simulink model "Pitoni_02"  (R2022b)
settings: Solver=VariableStepAuto  StartTime=0.0  StopTime=10  RelTol=1e-3
settings Model: Creator=Stefano  LastModifiedBy=stefanopanzieri
settings SolverCC: AlgebraicLoopSolver=TrustRegion
settings OptimizationCC: ReuseModelBlockBuffer=on
settings DebuggingCC: UnconnectedInputMsg=warning  UnconnectedOutputMsg=warning  UnconnectedLineMsg=warning
settings ModelReferenceCC: EnableRefExpFcnMdlSchedulingChecks=on
settings SFSimCC: CustomCodeUndefinedFunction=UseInterfaceOnly
settings RTWCC: DLArmComputeVersion=19.05

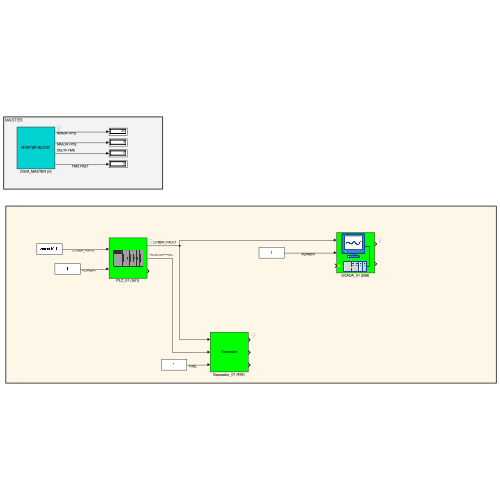
[thumbnail: Simulink's stored preview of the top-level diagram]
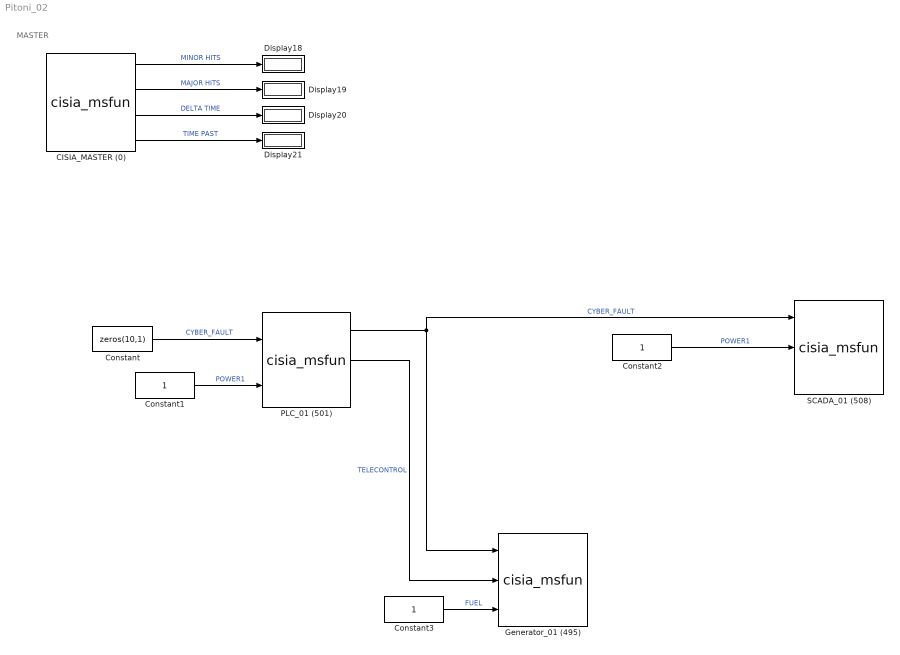
== system Pitoni_02 ==
  note: MASTER
  CISIA_MASTER (0) : M-S-Function  FunctionName=cisia_msfun  Parameters=Parameter1, Parameter2, Parameter3, resources, Parameter4, Parameter5, Parameter6, Parameter7, Parameter8, Parameter9,Parameter11  mask(S-function:msfcn_unit_delay){Parameter1='CISIA_MASTER', Parameter2=1, Parameter3='Pitoni', resources=off, Parameter4=on, Parameter5=off, Parameter6=off, Parameter7=off, Parameter8=0.001, Parameter9=off, Parameter11=on}
      mask prompts: Parameter1 "entity name"; Parameter2 "sampling time"; Parameter3 "project"; resources "Save status at each major hit"; Parameter4 "Show Operative Levels with colors"; Parameter5 "Load Entities from file"; Parameter6 "Load Start from Mask"; Parameter7 "Real Time"; Parameter8 "Real Time Hit (sec)"; Parameter9 "Skip saving"; Parameter11 "Show unconnected"
      mask help: This is a level-2 MATLAB file S-function which demonstrates CISIA entity
      mask Display: disp('MASTER BLOCK')
  Constant : Constant  Value=zeros(10,1)
  Constant1 : Constant
  Constant2 : Constant
  Constant3 : Constant
  Display{18..21} (4 alike) : Display
  Generator_01 (495) : M-S-Function  FunctionName=cisia_msfun  Parameters=Parameter1, Parameter2, Parameter3, resources, Parameter10, codeupdate, step_received, step_computed, dynamic_computed, step_sended, id_entity, id_project, id_type, name_type, color  mask(S-function:msfcn_unit_delay){Parameter1='Generator_01', Parameter2=1, Parameter3='', resources=|, Parameter10=off, codeupdate=off, step_received=|, step_computed=, dynamic_computed=, step_sended=|, id_entity=495, id_project=44, id_type=117, name_type=Generator, color=#FFFFFF}
      mask resources=|
      | *** INPUT RESOURCES ***
      | NUM_INPUTS 3
      | CYBER_FAULT (10)
      | TELECONTROL (1)
      | FUEL (1)
      |
      | *** STATE VARIABLES ***
      | NUM_VARIABLES 14
      | Operative_Level(NUMERIC)(1)(1)
      | Dos_attack(NUMERIC)(1)(0)
      | MITM_attack(NUMERIC)(1)(0)
      | Virus_Attack(NUMERIC)(1)(0)
      | Port_Scan_Attack(NUMERIC)(1)(0)
      | Cyber_Fault(NUMERIC_ARRAY)(10)(0  0  0  0  0  0  0  0  0  0)
      | BGP_hijacking(NUMERIC)(1)(0)
      | Mechanical_Fault(NUMERIC)(1)(0)
      | BotNet_Attack(NUMERIC)(1)(0)
      | Data_Corruption(NUMERIC)(1)(0)
      | SW_Change(NUMERIC)(1)(0)
      | Config_Change(NUMERIC)(1)(0)
      | Port_Saturation(NUMERIC)(1)(0)
      | Control_Fault(NUMERIC)(1)(0)
      |
      | *** OUTPUT RESOURCES ***
      | NUM_OUTPUTS 3
      | CYBER_FAULT (10)
      | POWER1 (1)
      | GENERATOR_QoS (1)
      mask step_received=|
      | Cyber_Fault=max(CYBER_FAULT, transpose([Dos_attack MITM_attack Virus_Attack Port_Scan_Attack  BGP_hijacking BotNet_Attack Data_Corruption SW_Change Config_Change Port_Saturation]));
      |
      | Control_Fault=max([1-TELECONTROL Mechanical_Fault Dos_attack min(0.5,max(Cyber_Fault))]);
      |
      | Operative_Level=min([1-max(Cyber_Fault) 1-Mechanical_Fault FUEL]);
      mask step_sended=|
      | POWER1 = Operative_Level
      | GENERATOR_QoS = Operative_Level
      | CYBER_FAULT=Cyber_Fault.*transpose([0 0 0.5 0.2 0 0 0 0 0 0]);
      mask prompts: Parameter1 "entity name"; Parameter2 "sampling time"; Parameter3 "project"; resources "input resources and state variables"; Parameter10 "Bring state variables to output"; codeupdate "update code from mask"
      mask help: This is a level-2 MATLAB file S-function which demonstrates CISIA entity
      mask DialogControl Container1 Prompt: All parameters
      mask Display: disp('Generator')
  PLC_01 (501) : M-S-Function  FunctionName=cisia_msfun  Parameters=Parameter1, Parameter2, Parameter3, resources, Parameter10, codeupdate, step_received, step_computed, dynamic_computed, step_sended, id_entity, id_project, id_type, name_type, color  mask(S-function:msfcn_unit_delay){Parameter1='PLC_01', Parameter2=1, Parameter3='', resources=|, Parameter10=off, codeupdate=off, step_received=|, step_computed=, dynamic_computed=, step_sended=|, id_entity=501, id_project=44, id_type=123, name_type=PLC, color=#FFFFFF}
      mask resources=|
      | *** INPUT RESOURCES ***
      | NUM_INPUTS 2
      | CYBER_FAULT (10)
      | POWER1 (1)
      |
      | *** STATE VARIABLES ***
      | NUM_VARIABLES 14
      | Operative_Level(NUMERIC)(1)(1)
      | Dos_attack(NUMERIC)(1)(0)
      | MITM_attack(NUMERIC)(1)(0)
      | Virus_Attack(NUMERIC)(1)(0)
      | Port_Scan_Attack(NUMERIC)(1)(0)
      | Cyber_Fault(NUMERIC_ARRAY)(10)(0  0  0  0  0  0  0  0  0  0)
      | BGP_hijacking(NUMERIC)(1)(0)
      | Mechanical_Fault(NUMERIC)(1)(0)
      | BotNet_Attack(NUMERIC)(1)(0)
      | Data_Corruption(NUMERIC)(1)(0)
      | SW_Change(NUMERIC)(1)(0)
      | Config_Change(NUMERIC)(1)(0)
      | Port_Saturation(NUMERIC)(1)(0)
      | Control_Fault(NUMERIC)(1)(0)
      |
      | *** OUTPUT RESOURCES ***
      | NUM_OUTPUTS 3
      | CYBER_FAULT (10)
      | TELECONTROL (1)
      | PLC_QoS (1)
      mask step_received=|
      | Cyber_Fault=max(CYBER_FAULT, transpose([Dos_attack MITM_attack Virus_Attack Port_Scan_Attack  BGP_hijacking BotNet_Attack Data_Corruption SW_Change Config_Change Port_Saturation]));
      |
      |
      | Control_Fault=max([Mechanical_Fault 1-POWER1 Dos_attack min(0.5,max(Cyber_Fault))]);
      |
      |
      |
      | Operative_Level=min([1-max(Cyber_Fault) 1-Mechanical_Fault 1-Control_Fault]);
      mask step_sended=|
      | CYBER_FAULT=Cyber_Fault.*transpose([0 0 0.5 0.2 0 0 0 0 0 0]);
      |
      | TELECONTROL=1-Control_Fault;
      | PLC_QoS=Operative_Level;
      mask prompts: Parameter1 "entity name"; Parameter2 "sampling time"; Parameter3 "project"; resources "input resources and state variables"; Parameter10 "Bring state variables to output"; codeupdate "update code from mask"
      mask help: This is a level-2 MATLAB file S-function which demonstrates CISIA entity
      mask DialogControl Container1 Prompt: All parameters
      mask Display: image('Icons/PLC.png')
  SCADA_01 (508) : M-S-Function  FunctionName=cisia_msfun  Parameters=Parameter1, Parameter2, Parameter3, resources, Parameter10, codeupdate, step_received, step_computed, dynamic_computed, step_sended, id_entity, id_project, id_type, name_type, color  mask(S-function:msfcn_unit_delay){Parameter1='SCADA_01', Parameter2=1, Parameter3='SistemiIoT', resources=|, Parameter10=off, codeupdate=off, step_received=|, step_computed=, dynamic_computed=, step_sended=|, id_entity=508, id_project=44, id_type=125, name_type=SCADA, color=#FFFFFF}
      mask resources=|
      | *** INPUT RESOURCES ***
      | NUM_INPUTS 3
      | CYBER_FAULT (10)
      | POWER1 (1)
      | PLC_QoS (1)
      |
      | *** STATE VARIABLES ***
      | NUM_VARIABLES 14
      | Operative_Level(NUMERIC)(1)(1)
      | Dos_attack(NUMERIC)(1)(0)
      | MITM_attack(NUMERIC)(1)(0)
      | Virus_Attack(NUMERIC)(1)(0)
      | Port_Scan_Attack(NUMERIC)(1)(0)
      | Cyber_Fault(NUMERIC_ARRAY)(10)(0  0  0  0  0  0  0  0  0  0)
      | BGP_hijacking(NUMERIC)(1)(0)
      | Mechanical_Fault(NUMERIC)(1)(0)
      | BotNet_Attack(NUMERIC)(1)(0)
      | Data_Corruption(NUMERIC)(1)(0)
      | SW_Change(NUMERIC)(1)(0)
      | Config_Change(NUMERIC)(1)(0)
      | Port_Saturation(NUMERIC)(1)(0)
      | Control_Fault(NUMERIC)(1)(0)
      |
      | *** OUTPUT RESOURCES ***
      | NUM_OUTPUTS 2
      | CYBER_FAULT (10)
      | SCADA_QoS (1)
      mask step_received=|
      | Cyber_Fault=max(CYBER_FAULT, transpose([Dos_attack MITM_attack Virus_Attack Port_Scan_Attack  BGP_hijacking BotNet_Attack Data_Corruption SW_Change Config_Change Port_Saturation]));
      |
      |
      | Control_Fault=max([Mechanical_Fault Dos_attack min(0.5,max(Cyber_Fault))]);
      |
      |
      |
      | %Operative_Level=min([1-max(Cyber_Fault) 1-Mechanical_Fault POWER1 PLC_QoS]);
      mask step_sended=|
      | SCADA_QoS=Operative_Level;
      |
      | CYBER_FAULT=Cyber_Fault.*transpose([0 0 0.5 0.2 0 0 0 0 0 0]);
      mask prompts: Parameter1 "entity name"; Parameter2 "sampling time"; Parameter3 "project"; resources "input resources and state variables"; Parameter10 "Bring state variables to output"; codeupdate "update code from mask"
      mask help: This is a level-2 MATLAB file S-function which demonstrates CISIA entity
      mask DialogControl Container1 Prompt: All parameters
      mask Display: image('Icons/SCADA.png');port_label('input',3,'\color{yellow}\spadesuit','texmode','on')
  wires:
  CISIA_MASTER (0)/1 -> Display18/1  "MINOR HITS"
  CISIA_MASTER (0)/2 -> Display19/1  "MAJOR HITS"
  CISIA_MASTER (0)/4 -> Display21/1  "TIME PAST"
  CISIA_MASTER (0)/3 -> Display20/1  "DELTA TIME"
  PLC_01 (501)/1 -> SCADA_01 (508)/1, Generator_01 (495)/1  "CYBER_FAULT"
  PLC_01 (501)/2 -> Generator_01 (495)/2  "TELECONTROL"
  Constant/1 -> PLC_01 (501)/1  "CYBER_FAULT"
  Constant1/1 -> PLC_01 (501)/2  "POWER1"
  Constant2/1 -> SCADA_01 (508)/2  "POWER1"
  Constant3/1 -> Generator_01 (495)/3  "FUEL"
